simulink model "saved3"  (R2018b)
settings: Solver=VariableStepAuto  StartTime=0.0  StopTime=10.0  RelTol=1e-3
libraries: simulink x95, powerlib x8, powerlib_meascontrol x2
(part 5 of 6)

== system saved3/离散化半成品/PSMS2/PMSM dq ==
  u1 : Inport
  u2 : Inport  Port=2
  torE : Inport  Port=3
  Gain : Gain  Gain=1/2
  Gain1 : Gain  Gain=1/2
  Integrator{,1..3} (4 alike) : Integrator
  MATLAB Function : MATLAB Function  TreatAsAtomicUnit=on
  MATLAB Function1 : MATLAB Function  TreatAsAtomicUnit=on
  Sum : Sum  Inputs=|++
  角度增速测试 : simulink/Sources/Ramp  slope=0  start=0  InitialOutput=0
  i1 : Outport
  i2 : Outport  Port=2
  w : Outport  Port=3
  the : Outport  Port=4
  wires:
  MATLAB Function1/1(dw) -> Integrator2/1
  u1/1 -> Gain/1
  MATLAB Function/2(di2) -> Integrator1/1
  MATLAB Function/1(di1) -> Integrator/1
  Integrator/1 -> i1/1, MATLAB Function1/1(i1), MATLAB Function/3(i1)
  Integrator1/1 -> MATLAB Function/4(i2), MATLAB Function1/2(i2), i2/1
  torE/1 -> MATLAB Function1/4(torE)
  Gain/1 -> MATLAB Function/1(u1)
  u2/1 -> Gain1/1
  Gain1/1 -> MATLAB Function/2(u2)
  Integrator3/1 -> the/1
  Integrator2/1 -> Sum/1, MATLAB Function1/3(w), MATLAB Function/5(w), w/1
  Sum/1 -> Integrator3/1
  角度增速测试/1 -> Sum/2

== system saved3/离散化半成品/PSMS3/PMSM dq ==
  u1 : Inport
  u2 : Inport  Port=2
  torE : Inport  Port=3
  Gain : Gain  Gain=1/2
  Gain1 : Gain  Gain=1/2
  Integrator{,1..3} (4 alike) : Integrator
  MATLAB Function : MATLAB Function  TreatAsAtomicUnit=on
  MATLAB Function1 : MATLAB Function  TreatAsAtomicUnit=on
  Sum : Sum  Inputs=|++
  角度增速测试 : simulink/Sources/Ramp  slope=0  start=0  InitialOutput=0
  i1 : Outport
  i2 : Outport  Port=2
  w : Outport  Port=3
  the : Outport  Port=4
  wires:
  MATLAB Function1/1(dw) -> Integrator2/1
  u1/1 -> Gain/1
  MATLAB Function/2(di2) -> Integrator1/1
  MATLAB Function/1(di1) -> Integrator/1
  Integrator/1 -> i1/1, MATLAB Function1/1(i1), MATLAB Function/3(i1)
  Integrator1/1 -> MATLAB Function/4(i2), MATLAB Function1/2(i2), i2/1
  torE/1 -> MATLAB Function1/4(torE)
  Gain/1 -> MATLAB Function/1(u1)
  u2/1 -> Gain1/1
  Gain1/1 -> MATLAB Function/2(u2)
  Integrator3/1 -> the/1
  Integrator2/1 -> Sum/1, MATLAB Function1/3(w), MATLAB Function/5(w), w/1
  Sum/1 -> Integrator3/1
  角度增速测试/1 -> Sum/2

== system saved3/离散化半成品/Subsystem/电流采样 ==
  <Stator current is_a (A)> : Inport
  <Stator current is_b (A)> : Inport  Port=2
  <Stator current is_c (A)> : Inport  Port=3
  A/D转换 10KHz2 : MATLAB Function  TreatAsAtomicUnit=on  SystemSampleTime=1e-4
  A/D转换 10KHz3 : MATLAB Function  TreatAsAtomicUnit=on  SystemSampleTime=1e-4
  A/D转换 10KHz4 : MATLAB Function  TreatAsAtomicUnit=on  SystemSampleTime=1e-4
  Scope : Scope  NumInputPorts=3
  Sum1 : Sum  Inputs=|++
  Sum2 : Sum  Inputs=|++
  Sum3 : Sum  Inputs=|+-
  一阶滤波器40kHz1 : MATLAB Function  Commented=on  TreatAsAtomicUnit=on  SystemSampleTime=2.5e-5
  一阶滤波器40kHz2 : MATLAB Function  Commented=on  TreatAsAtomicUnit=on  SystemSampleTime=2.5e-5
  一阶滤波器40kHz3 : MATLAB Function  Commented=on  TreatAsAtomicUnit=on  SystemSampleTime=2.5e-5
  噪声 ia : simulink/Sources/Band-Limited White Noise  Cov=1e-7  Ts=1e-4  seed=[1]
  噪声 ib : simulink/Sources/Band-Limited White Noise  Cov=1e-7  Ts=1e-4  seed=[2]
  噪声 ic : simulink/Sources/Band-Limited White Noise  Cov=1e-7  Ts=1e-4  seed=[3]
  ia : Outport
  ib : Outport  Port=2
  ic : Outport  Port=3
  wires:
  Sum1/1 -> A/D转换 10KHz2/1(u)
  Sum2/1 -> A/D转换 10KHz3/1(u)
  Sum3/1 -> A/D转换 10KHz4/1(u)
  <Stator current is_b (A)>/1 -> Sum2/1
  <Stator current is_c (A)>/1 -> Sum3/1
  <Stator current is_a (A)>/1 -> Sum1/1
  A/D转换 10KHz2/1(y) -> Scope/1, ia/1
  A/D转换 10KHz3/1(y) -> Scope/2, ib/1
  A/D转换 10KHz4/1(y) -> Scope/3, ic/1
  噪声 ia/1 -> Sum1/2
  噪声 ic/1 -> Sum3/2
  噪声 ib/1 -> Sum2/2

== system saved3/离散化半成品/controller/方波注入 ==
  Constant2 : Constant  Value=0.5
  Gain11 : Gain  Gain=8
  Pulse Generator2 : DiscretePulseGenerator  PulseType=Time based  Period=1e-3  PulseWidth=50
  Sum4 : Sum  Inputs=|+-
  Out1 : Outport
  wires:
  Pulse Generator2/1 -> Sum4/1
  Sum4/1 -> Gain11/1
  Constant2/1 -> Sum4/2
  Gain11/1 -> Out1/1

== system saved3/离散化半成品/controller1/方波注入 ==
  Constant2 : Constant  Value=0.5
  Gain11 : Gain  Gain=8
  Pulse Generator2 : DiscretePulseGenerator  PulseType=Time based  Period=1e-3  PulseWidth=50
  Sum4 : Sum  Inputs=|+-
  Out1 : Outport
  wires:
  Pulse Generator2/1 -> Sum4/1
  Sum4/1 -> Gain11/1
  Constant2/1 -> Sum4/2
  Gain11/1 -> Out1/1

== system saved3/离散化半成品/controller2/方波注入 ==
  Constant2 : Constant  Value=0.5
  Gain11 : Gain  Gain=8
  Pulse Generator2 : DiscretePulseGenerator  PulseType=Time based  Period=1e-3  PulseWidth=50
  Sum4 : Sum  Inputs=|+-
  Out1 : Outport
  wires:
  Pulse Generator2/1 -> Sum4/1
  Sum4/1 -> Gain11/1
  Constant2/1 -> Sum4/2
  Gain11/1 -> Out1/1

== system saved3/离散化半成品/controller3/方波注入 ==
  Constant2 : Constant  Value=0.5
  Gain11 : Gain  Gain=8
  Pulse Generator2 : DiscretePulseGenerator  PulseType=Time based  Period=1e-3  PulseWidth=50
  Sum4 : Sum  Inputs=|+-
  Out1 : Outport
  wires:
  Pulse Generator2/1 -> Sum4/1
  Sum4/1 -> Gain11/1
  Constant2/1 -> Sum4/2
  Gain11/1 -> Out1/1

== system saved3/离散化半成品/current seperator/电流采样 ==
  <Stator current is_a (A)> : Inport
  <Stator current is_b (A)> : Inport  Port=2
  <Stator current is_c (A)> : Inport  Port=3
  A/D转换 10KHz2 : MATLAB Function  TreatAsAtomicUnit=on  SystemSampleTime=1e-4
  A/D转换 10KHz3 : MATLAB Function  TreatAsAtomicUnit=on  SystemSampleTime=1e-4
  A/D转换 10KHz4 : MATLAB Function  TreatAsAtomicUnit=on  SystemSampleTime=1e-4
  Scope : Scope  NumInputPorts=3
  Sum1 : Sum  Inputs=|++
  Sum2 : Sum  Inputs=|++
  Sum3 : Sum  Inputs=|+-
  噪声 ia : simulink/Sources/Band-Limited White Noise  Cov=1e-7  Ts=1e-4  seed=[1]
  噪声 ib : simulink/Sources/Band-Limited White Noise  Cov=1e-7  Ts=1e-4  seed=[2]
  噪声 ic : simulink/Sources/Band-Limited White Noise  Cov=1e-7  Ts=1e-4  seed=[3]
  ia : Outport
  ib : Outport  Port=2
  ic : Outport  Port=3
  wires:
  Sum1/1 -> A/D转换 10KHz2/1(u)
  Sum2/1 -> A/D转换 10KHz3/1(u)
  Sum3/1 -> A/D转换 10KHz4/1(u)
  <Stator current is_b (A)>/1 -> Sum2/1
  <Stator current is_c (A)>/1 -> Sum3/1
  <Stator current is_a (A)>/1 -> Sum1/1
  A/D转换 10KHz2/1(y) -> Scope/1, ia/1
  A/D转换 10KHz3/1(y) -> Scope/2, ib/1
  A/D转换 10KHz4/1(y) -> Scope/3, ic/1
  噪声 ia/1 -> Sum1/2
  噪声 ic/1 -> Sum3/2
  噪声 ib/1 -> Sum2/2

== system saved3/离散化半成品/current seperator/电流采样1 ==
  <Stator current is_a (A)> : Inport
  <Stator current is_b (A)> : Inport  Port=2
  <Stator current is_c (A)> : Inport  Port=3
  A/D转换 10KHz2 : MATLAB Function  TreatAsAtomicUnit=on  SystemSampleTime=1e-4
  A/D转换 10KHz3 : MATLAB Function  TreatAsAtomicUnit=on  SystemSampleTime=1e-4
  A/D转换 10KHz4 : MATLAB Function  TreatAsAtomicUnit=on  SystemSampleTime=1e-4
  Scope : Scope  NumInputPorts=3
  Sum1 : Sum  Inputs=|++
  Sum2 : Sum  Inputs=|++
  Sum3 : Sum  Inputs=|+-
  噪声 ia : simulink/Sources/Band-Limited White Noise  Cov=1e-7  Ts=1e-4  seed=[1]
  噪声 ib : simulink/Sources/Band-Limited White Noise  Cov=1e-7  Ts=1e-4  seed=[2]
  噪声 ic : simulink/Sources/Band-Limited White Noise  Cov=1e-7  Ts=1e-4  seed=[3]
  ia : Outport
  ib : Outport  Port=2
  ic : Outport  Port=3
  wires:
  Sum1/1 -> A/D转换 10KHz2/1(u)
  Sum2/1 -> A/D转换 10KHz3/1(u)
  Sum3/1 -> A/D转换 10KHz4/1(u)
  <Stator current is_b (A)>/1 -> Sum2/1
  <Stator current is_c (A)>/1 -> Sum3/1
  <Stator current is_a (A)>/1 -> Sum1/1
  A/D转换 10KHz2/1(y) -> Scope/1, ia/1
  A/D转换 10KHz3/1(y) -> Scope/2, ib/1
  A/D转换 10KHz4/1(y) -> Scope/3, ic/1
  噪声 ia/1 -> Sum1/2
  噪声 ic/1 -> Sum3/2
  噪声 ib/1 -> Sum2/2

== system saved3/离散化半成品/w estimater/Subsystem ==
  ua : Inport
  ub : Inport  Port=2
  ia : Inport  Port=3
  ib : Inport  Port=4
  1/Lm1 : Gain  Gain=1/1.2e-3
  1/Lm2 : Gain  Gain=1/1.2e-3
  Gain : Gain
  Gain1 : Gain
  Integrator : Integrator
  Integrator1 : Integrator
  PID Controller : simulink/Continuous/PID Controller  Controller=PID  Form=Parallel  TimeDomain=Continuous-time  SampleTime=-1  IntegratorMethod=Forward Euler  FilterMethod=Forward Euler  ControllerParametersSource=internal  P=10  I=10  D=1  UseFilter=on  N=100  TunerSelectOption=Transfer Function Based (PID Tuner App)  InitialConditionSource=internal  InitialConditionForIntegrator=0  InitialConditionForFilter=0  DifferentiatorICPrevScaledInput=0  ExternalReset=none  TrackingMode=off  Kt=1  LimitOutput=off  UpperSaturationLimit=inf  LowerSaturationLimit=-inf  LinearizeAsGain=on  AntiWindupMode=none  Kb=1  POutMin=[]  POutMax=[]  IOutMin=[]  IOutMax=[]  DOutMin=[]  DOutMax=[]  NOutMin=[]  NOutMax=[]  SumOutMin=[]  SumOutMax=[]  SaturationOutMin=[]  SaturationOutMax=[]  PParamMin=[]  PParamMax=[]  IParamMin=[]  IParamMax=[]  DParamMin=[]  DParamMax=[]  NParamMin=[]  NParamMax=[]  KbParamMin=[]  KbParamMax=[]  KtParamMin=[]  KtParamMax=[]  KbOutMin=[]  KbOutMax=[]  KtOutMin=[]  KtOutMax=[]  IntegratorOutMin=[]  IntegratorOutMax=[]  FilterOutMin=[]  FilterOutMax=[]  SumI1OutMin=[]  SumI1OutMax=[]  SumI2OutMin=[]  SumI2OutMax=[]  SumI3OutMin=[]  SumI3OutMax=[]  SumI4OutMin=[]  SumI4OutMax=[]  SumDOutMin=[]  SumDOutMax=[]  DifferentiatorOutMin=[]  DifferentiatorOutMax=[]  FilterDiffOutCoefMin=[]  FilterDiffOutCoefMax=[]  ReciprocalOutMin=[]  ReciprocalOutMax=[]  SumDenOutMin=[]  SumDenOutMax=[]  SumNumOutMin=[]  SumNumOutMax=[]  DivideOutMin=[]  DivideOutMax=[]  IntegratorContinuousStateAttributes=''  IntegratorStateMustResolveToSignalObject=off  IntegratorRTWStateStorageClass=Auto  FilterContinuousStateAttributes=''  FilterStateMustResolveToSignalObject=off  FilterRTWStateStorageClass=Auto  ParallelPVariant=InternalParameters  IdealPVariant=Disabled  IVariant=InternalParameters  DVariant=InternalParameters  IntegratorVariant=Continuous  SatVariant=Disabled  AWVariant=Passthrough  PCopyVariant=Disabled  TRVariant=Disabled  FdbkBlocksVariant=Forward  IdealPFdbkVariant=Disabled  SatFdbkVariant=Disabled  DerivativeFilterVariant=ContFilter  NVariant=InternalParameters  NCopyVariant=Disabled  FilterICVariant=InternalICsFilter  IntegratorICVariant=InternalICs  ExternalResetVariant=Disabled  TRSumVariant=Passthrough  SumFdbkVariant=Disabled  SumVariant=Sum_PID
  PID Controller1 : simulink/Continuous/PID Controller  Controller=PID  Form=Parallel  TimeDomain=Continuous-time  SampleTime=-1  IntegratorMethod=Forward Euler  FilterMethod=Forward Euler  ControllerParametersSource=internal  P=3  I=10  D=1  UseFilter=on  N=100  TunerSelectOption=Transfer Function Based (PID Tuner App)  InitialConditionSource=internal  InitialConditionForIntegrator=0  InitialConditionForFilter=0  DifferentiatorICPrevScaledInput=0  ExternalReset=none  TrackingMode=off  Kt=1  LimitOutput=off  UpperSaturationLimit=inf  LowerSaturationLimit=-inf  LinearizeAsGain=on  AntiWindupMode=none  Kb=1  POutMin=[]  POutMax=[]  IOutMin=[]  IOutMax=[]  DOutMin=[]  DOutMax=[]  NOutMin=[]  NOutMax=[]  SumOutMin=[]  SumOutMax=[]  SaturationOutMin=[]  SaturationOutMax=[]  PParamMin=[]  PParamMax=[]  IParamMin=[]  IParamMax=[]  DParamMin=[]  DParamMax=[]  NParamMin=[]  NParamMax=[]  KbParamMin=[]  KbParamMax=[]  KtParamMin=[]  KtParamMax=[]  KbOutMin=[]  KbOutMax=[]  KtOutMin=[]  KtOutMax=[]  IntegratorOutMin=[]  IntegratorOutMax=[]  FilterOutMin=[]  FilterOutMax=[]  SumI1OutMin=[]  SumI1OutMax=[]  SumI2OutMin=[]  SumI2OutMax=[]  SumI3OutMin=[]  SumI3OutMax=[]  SumI4OutMin=[]  SumI4OutMax=[]  SumDOutMin=[]  SumDOutMax=[]  DifferentiatorOutMin=[]  DifferentiatorOutMax=[]  FilterDiffOutCoefMin=[]  FilterDiffOutCoefMax=[]  ReciprocalOutMin=[]  ReciprocalOutMax=[]  SumDenOutMin=[]  SumDenOutMax=[]  SumNumOutMin=[]  SumNumOutMax=[]  DivideOutMin=[]  DivideOutMax=[]  IntegratorContinuousStateAttributes=''  IntegratorStateMustResolveToSignalObject=off  IntegratorRTWStateStorageClass=Auto  FilterContinuousStateAttributes=''  FilterStateMustResolveToSignalObject=off  FilterRTWStateStorageClass=Auto  ParallelPVariant=InternalParameters  IdealPVariant=Disabled  IVariant=InternalParameters  DVariant=InternalParameters  IntegratorVariant=Continuous  SatVariant=Disabled  AWVariant=Passthrough  PCopyVariant=Disabled  TRVariant=Disabled  FdbkBlocksVariant=Forward  IdealPFdbkVariant=Disabled  SatFdbkVariant=Disabled  DerivativeFilterVariant=ContFilter  NVariant=InternalParameters  NCopyVariant=Disabled  FilterICVariant=InternalICsFilter  IntegratorICVariant=InternalICs  ExternalResetVariant=Disabled  TRSumVariant=Passthrough  SumFdbkVariant=Disabled  SumVariant=Sum_PID
  R1 : Gain  Gain=0.1
  R2 : Gain  Gain=0.1
  Scope : Scope  NumInputPorts=2
  Scope1 : Scope  NumInputPorts=2
  Scope2 : Scope  NumInputPorts=2
  Sum : Sum  Inputs=|+-
  Sum1 : Sum  Inputs=++-
  Sum2 : Sum  Inputs=|+-
  Sum3 : Sum  Inputs=++-
  Ea : Outport
  Eb : Outport  Port=2
  wires:
  Sum/1 -> Gain1/1
  R1/1 -> Sum1/3
  Integrator/1 -> Scope2/2, Sum/2, R1/1
  Sum1/1 -> 1/Lm1/1
  1/Lm1/1 -> Integrator/1
  ua/1 -> Sum1/1
  ia/1 -> Scope2/1, Sum/1
  ib/1 -> Scope1/1, Sum2/1
  ub/1 -> Sum3/1
  Sum2/1 -> Gain/1
  1/Lm2/1 -> Integrator1/1
  R2/1 -> Sum3/3
  Sum3/1 -> 1/Lm2/1
  Integrator1/1 -> Sum2/2, Scope1/2, R2/1
  Gain/1 -> PID Controller1/1
  Gain1/1 -> PID Controller/1
  PID Controller1/1 -> Scope/2, Eb/1, Sum3/2
  PID Controller/1 -> Ea/1, Scope/1, Sum1/2

== system saved3/离散化半成品/w estimater/锁相环 ==
  cos : Inport
  sin : Inport  Port=2
  Constant : Constant  Value=0
  Cos : Trigonometry  Operator=cos
  Gain : Gain  Gain=-1
  Integrator2 : Integrator
  PID Controller : simulink/Continuous/PID Controller  Controller=PID  Form=Parallel  TimeDomain=Continuous-time  SampleTime=-1  IntegratorMethod=Forward Euler  FilterMethod=Forward Euler  ControllerParametersSource=internal  P=40  I=5000  D=0  UseFilter=on  N=100  TunerSelectOption=Transfer Function Based (PID Tuner App)  InitialConditionSource=internal  InitialConditionForIntegrator=0  InitialConditionForFilter=0  DifferentiatorICPrevScaledInput=0  ExternalReset=none  TrackingMode=off  Kt=1  LimitOutput=off  UpperSaturationLimit=inf  LowerSaturationLimit=-inf  LinearizeAsGain=on  AntiWindupMode=none  Kb=1  POutMin=[]  POutMax=[]  IOutMin=[]  IOutMax=[]  DOutMin=[]  DOutMax=[]  NOutMin=[]  NOutMax=[]  SumOutMin=[]  SumOutMax=[]  SaturationOutMin=[]  SaturationOutMax=[]  PParamMin=[]  PParamMax=[]  IParamMin=[]  IParamMax=[]  DParamMin=[]  DParamMax=[]  NParamMin=[]  NParamMax=[]  KbParamMin=[]  KbParamMax=[]  KtParamMin=[]  KtParamMax=[]  KbOutMin=[]  KbOutMax=[]  KtOutMin=[]  KtOutMax=[]  IntegratorOutMin=[]  IntegratorOutMax=[]  FilterOutMin=[]  FilterOutMax=[]  SumI1OutMin=[]  SumI1OutMax=[]  SumI2OutMin=[]  SumI2OutMax=[]  SumI3OutMin=[]  SumI3OutMax=[]  SumI4OutMin=[]  SumI4OutMax=[]  SumDOutMin=[]  SumDOutMax=[]  DifferentiatorOutMin=[]  DifferentiatorOutMax=[]  FilterDiffOutCoefMin=[]  FilterDiffOutCoefMax=[]  ReciprocalOutMin=[]  ReciprocalOutMax=[]  SumDenOutMin=[]  SumDenOutMax=[]  SumNumOutMin=[]  SumNumOutMax=[]  DivideOutMin=[]  DivideOutMax=[]  IntegratorContinuousStateAttributes=''  IntegratorStateMustResolveToSignalObject=off  IntegratorRTWStateStorageClass=Auto  FilterContinuousStateAttributes=''  FilterStateMustResolveToSignalObject=off  FilterRTWStateStorageClass=Auto  ParallelPVariant=InternalParameters  IdealPVariant=Disabled  IVariant=InternalParameters  DVariant=InternalParameters  IntegratorVariant=Continuous  SatVariant=Disabled  AWVariant=Passthrough  PCopyVariant=Disabled  TRVariant=Disabled  FdbkBlocksVariant=Forward  IdealPFdbkVariant=Disabled  SatFdbkVariant=Disabled  DerivativeFilterVariant=ContFilter  NVariant=InternalParameters  NCopyVariant=Disabled  FilterICVariant=InternalICsFilter  IntegratorICVariant=InternalICs  ExternalResetVariant=Disabled  TRSumVariant=Passthrough  SumFdbkVariant=Disabled  SumVariant=Sum_PID
  Product : Product
  Product1 : Product
  Saturation : Saturate  UpperLimit=500  LowerLimit=-500
  Scope : Scope
  Sin : Trigonometry
  Sum : Sum  Inputs=+-
  Sum1 : Sum  Inputs=|+-
  Transfer Fcn : TransferFcn  Numerator=[100]  Denominator=[1 100]
  Transfer Fcn1 : TransferFcn  Numerator=[100]  Denominator=[1 100]
  Transfer Fcn2 : TransferFcn  Numerator=[100]  Denominator=[1 100]
  we : Outport
  the : Outport  Port=2
  wires:
  cos/1 -> Transfer Fcn1/1
  Cos/1 -> Product1/2
  Product1/1 -> Sum/1
  Product/1 -> Sum/2
  Sin/1 -> Product/2
  Sum/1 -> PID Controller/1, Scope/1
  Integrator2/1 -> Sin/1, Cos/1, Sum1/1
  PID Controller/1 -> Saturation/1, Integrator2/1
  Transfer Fcn/1 -> we/1
  Sum1/1 -> the/1
  Constant/1 -> Sum1/2
  sin/1 -> Transfer Fcn2/1
  Gain/1 -> Product/1
  Saturation/1 -> Transfer Fcn/1
  Transfer Fcn1/1 -> Product1/1
  Transfer Fcn2/1 -> Gain/1

== system saved3/离散化半成品/w estimater1/Subsystem1 ==
  ua : Inport
  ub : Inport  Port=2
  ia : Inport  Port=3
  ib : Inport  Port=4
  1/Lm1 : Gain  Gain=1/1.2e-3
  1/Lm2 : Gain  Gain=1/1.2e-3
  Gain : Gain
  Gain1 : Gain
  Integrator : Integrator
  Integrator1 : Integrator
  PID Controller : simulink/Continuous/PID Controller  Controller=PID  Form=Parallel  TimeDomain=Continuous-time  SampleTime=-1  IntegratorMethod=Forward Euler  FilterMethod=Forward Euler  ControllerParametersSource=internal  P=10  I=10  D=1  UseFilter=on  N=100  TunerSelectOption=Transfer Function Based (PID Tuner App)  InitialConditionSource=internal  InitialConditionForIntegrator=0  InitialConditionForFilter=0  DifferentiatorICPrevScaledInput=0  ExternalReset=none  TrackingMode=off  Kt=1  LimitOutput=off  UpperSaturationLimit=inf  LowerSaturationLimit=-inf  LinearizeAsGain=on  AntiWindupMode=none  Kb=1  POutMin=[]  POutMax=[]  IOutMin=[]  IOutMax=[]  DOutMin=[]  DOutMax=[]  NOutMin=[]  NOutMax=[]  SumOutMin=[]  SumOutMax=[]  SaturationOutMin=[]  SaturationOutMax=[]  PParamMin=[]  PParamMax=[]  IParamMin=[]  IParamMax=[]  DParamMin=[]  DParamMax=[]  NParamMin=[]  NParamMax=[]  KbParamMin=[]  KbParamMax=[]  KtParamMin=[]  KtParamMax=[]  KbOutMin=[]  KbOutMax=[]  KtOutMin=[]  KtOutMax=[]  IntegratorOutMin=[]  IntegratorOutMax=[]  FilterOutMin=[]  FilterOutMax=[]  SumI1OutMin=[]  SumI1OutMax=[]  SumI2OutMin=[]  SumI2OutMax=[]  SumI3OutMin=[]  SumI3OutMax=[]  SumI4OutMin=[]  SumI4OutMax=[]  SumDOutMin=[]  SumDOutMax=[]  DifferentiatorOutMin=[]  DifferentiatorOutMax=[]  FilterDiffOutCoefMin=[]  FilterDiffOutCoefMax=[]  ReciprocalOutMin=[]  ReciprocalOutMax=[]  SumDenOutMin=[]  SumDenOutMax=[]  SumNumOutMin=[]  SumNumOutMax=[]  DivideOutMin=[]  DivideOutMax=[]  IntegratorContinuousStateAttributes=''  IntegratorStateMustResolveToSignalObject=off  IntegratorRTWStateStorageClass=Auto  FilterContinuousStateAttributes=''  FilterStateMustResolveToSignalObject=off  FilterRTWStateStorageClass=Auto  ParallelPVariant=InternalParameters  IdealPVariant=Disabled  IVariant=InternalParameters  DVariant=InternalParameters  IntegratorVariant=Continuous  SatVariant=Disabled  AWVariant=Passthrough  PCopyVariant=Disabled  TRVariant=Disabled  FdbkBlocksVariant=Forward  IdealPFdbkVariant=Disabled  SatFdbkVariant=Disabled  DerivativeFilterVariant=ContFilter  NVariant=InternalParameters  NCopyVariant=Disabled  FilterICVariant=InternalICsFilter  IntegratorICVariant=InternalICs  ExternalResetVariant=Disabled  TRSumVariant=Passthrough  SumFdbkVariant=Disabled  SumVariant=Sum_PID
  PID Controller1 : simulink/Continuous/PID Controller  Controller=PID  Form=Parallel  TimeDomain=Continuous-time  SampleTime=-1  IntegratorMethod=Forward Euler  FilterMethod=Forward Euler  ControllerParametersSource=internal  P=3  I=10  D=1  UseFilter=on  N=100  TunerSelectOption=Transfer Function Based (PID Tuner App)  InitialConditionSource=internal  InitialConditionForIntegrator=0  InitialConditionForFilter=0  DifferentiatorICPrevScaledInput=0  ExternalReset=none  TrackingMode=off  Kt=1  LimitOutput=off  UpperSaturationLimit=inf  LowerSaturationLimit=-inf  LinearizeAsGain=on  AntiWindupMode=none  Kb=1  POutMin=[]  POutMax=[]  IOutMin=[]  IOutMax=[]  DOutMin=[]  DOutMax=[]  NOutMin=[]  NOutMax=[]  SumOutMin=[]  SumOutMax=[]  SaturationOutMin=[]  SaturationOutMax=[]  PParamMin=[]  PParamMax=[]  IParamMin=[]  IParamMax=[]  DParamMin=[]  DParamMax=[]  NParamMin=[]  NParamMax=[]  KbParamMin=[]  KbParamMax=[]  KtParamMin=[]  KtParamMax=[]  KbOutMin=[]  KbOutMax=[]  KtOutMin=[]  KtOutMax=[]  IntegratorOutMin=[]  IntegratorOutMax=[]  FilterOutMin=[]  FilterOutMax=[]  SumI1OutMin=[]  SumI1OutMax=[]  SumI2OutMin=[]  SumI2OutMax=[]  SumI3OutMin=[]  SumI3OutMax=[]  SumI4OutMin=[]  SumI4OutMax=[]  SumDOutMin=[]  SumDOutMax=[]  DifferentiatorOutMin=[]  DifferentiatorOutMax=[]  FilterDiffOutCoefMin=[]  FilterDiffOutCoefMax=[]  ReciprocalOutMin=[]  ReciprocalOutMax=[]  SumDenOutMin=[]  SumDenOutMax=[]  SumNumOutMin=[]  SumNumOutMax=[]  DivideOutMin=[]  DivideOutMax=[]  IntegratorContinuousStateAttributes=''  IntegratorStateMustResolveToSignalObject=off  IntegratorRTWStateStorageClass=Auto  FilterContinuousStateAttributes=''  FilterStateMustResolveToSignalObject=off  FilterRTWStateStorageClass=Auto  ParallelPVariant=InternalParameters  IdealPVariant=Disabled  IVariant=InternalParameters  DVariant=InternalParameters  IntegratorVariant=Continuous  SatVariant=Disabled  AWVariant=Passthrough  PCopyVariant=Disabled  TRVariant=Disabled  FdbkBlocksVariant=Forward  IdealPFdbkVariant=Disabled  SatFdbkVariant=Disabled  DerivativeFilterVariant=ContFilter  NVariant=InternalParameters  NCopyVariant=Disabled  FilterICVariant=InternalICsFilter  IntegratorICVariant=InternalICs  ExternalResetVariant=Disabled  TRSumVariant=Passthrough  SumFdbkVariant=Disabled  SumVariant=Sum_PID
  R1 : Gain  Gain=0.1
  R2 : Gain  Gain=0.1
  Scope : Scope  NumInputPorts=2
  Scope1 : Scope  NumInputPorts=2
  Scope2 : Scope  NumInputPorts=2
  Sum : Sum  Inputs=|+-
  Sum1 : Sum  Inputs=++-
  Sum2 : Sum  Inputs=|+-
  Sum3 : Sum  Inputs=++-
  Ea : Outport
  Eb : Outport  Port=2
  wires:
  Sum/1 -> Gain1/1
  R1/1 -> Sum1/3
  Integrator/1 -> Scope2/2, Sum/2, R1/1
  Sum1/1 -> 1/Lm1/1
  1/Lm1/1 -> Integrator/1
  ua/1 -> Sum1/1
  ia/1 -> Scope2/1, Sum/1
  ib/1 -> Scope1/1, Sum2/1
  ub/1 -> Sum3/1
  Sum2/1 -> Gain/1
  1/Lm2/1 -> Integrator1/1
  R2/1 -> Sum3/3
  Sum3/1 -> 1/Lm2/1
  Integrator1/1 -> Sum2/2, Scope1/2, R2/1
  Gain/1 -> PID Controller1/1
  Gain1/1 -> PID Controller/1
  PID Controller1/1 -> Scope/2, Eb/1, Sum3/2
  PID Controller/1 -> Ea/1, Scope/1, Sum1/2

== system saved3/离散化半成品/w estimater1/锁相环1 ==
  cos : Inport
  sin : Inport  Port=2
  Constant : Constant  Value=0
  Cos : Trigonometry  Operator=cos
  Gain : Gain  Gain=-1
  Integrator2 : Integrator
  PID Controller : simulink/Continuous/PID Controller  Controller=PID  Form=Parallel  TimeDomain=Continuous-time  SampleTime=-1  IntegratorMethod=Forward Euler  FilterMethod=Forward Euler  ControllerParametersSource=internal  P=40  I=5000  D=0  UseFilter=on  N=100  TunerSelectOption=Transfer Function Based (PID Tuner App)  InitialConditionSource=internal  InitialConditionForIntegrator=0  InitialConditionForFilter=0  DifferentiatorICPrevScaledInput=0  ExternalReset=none  TrackingMode=off  Kt=1  LimitOutput=off  UpperSaturationLimit=inf  LowerSaturationLimit=-inf  LinearizeAsGain=on  AntiWindupMode=none  Kb=1  POutMin=[]  POutMax=[]  IOutMin=[]  IOutMax=[]  DOutMin=[]  DOutMax=[]  NOutMin=[]  NOutMax=[]  SumOutMin=[]  SumOutMax=[]  SaturationOutMin=[]  SaturationOutMax=[]  PParamMin=[]  PParamMax=[]  IParamMin=[]  IParamMax=[]  DParamMin=[]  DParamMax=[]  NParamMin=[]  NParamMax=[]  KbParamMin=[]  KbParamMax=[]  KtParamMin=[]  KtParamMax=[]  KbOutMin=[]  KbOutMax=[]  KtOutMin=[]  KtOutMax=[]  IntegratorOutMin=[]  IntegratorOutMax=[]  FilterOutMin=[]  FilterOutMax=[]  SumI1OutMin=[]  SumI1OutMax=[]  SumI2OutMin=[]  SumI2OutMax=[]  SumI3OutMin=[]  SumI3OutMax=[]  SumI4OutMin=[]  SumI4OutMax=[]  SumDOutMin=[]  SumDOutMax=[]  DifferentiatorOutMin=[]  DifferentiatorOutMax=[]  FilterDiffOutCoefMin=[]  FilterDiffOutCoefMax=[]  ReciprocalOutMin=[]  ReciprocalOutMax=[]  SumDenOutMin=[]  SumDenOutMax=[]  SumNumOutMin=[]  SumNumOutMax=[]  DivideOutMin=[]  DivideOutMax=[]  IntegratorContinuousStateAttributes=''  IntegratorStateMustResolveToSignalObject=off  IntegratorRTWStateStorageClass=Auto  FilterContinuousStateAttributes=''  FilterStateMustResolveToSignalObject=off  FilterRTWStateStorageClass=Auto  ParallelPVariant=InternalParameters  IdealPVariant=Disabled  IVariant=InternalParameters  DVariant=InternalParameters  IntegratorVariant=Continuous  SatVariant=Disabled  AWVariant=Passthrough  PCopyVariant=Disabled  TRVariant=Disabled  FdbkBlocksVariant=Forward  IdealPFdbkVariant=Disabled  SatFdbkVariant=Disabled  DerivativeFilterVariant=ContFilter  NVariant=InternalParameters  NCopyVariant=Disabled  FilterICVariant=InternalICsFilter  IntegratorICVariant=InternalICs  ExternalResetVariant=Disabled  TRSumVariant=Passthrough  SumFdbkVariant=Disabled  SumVariant=Sum_PID
  Product : Product
  Product1 : Product
  Saturation : Saturate  UpperLimit=500  LowerLimit=-500
  Scope : Scope
  Sin : Trigonometry
  Sum : Sum  Inputs=+-
  Sum1 : Sum  Inputs=|+-
  Transfer Fcn : TransferFcn  Numerator=[100]  Denominator=[1 100]
  Transfer Fcn1 : TransferFcn  Numerator=[100]  Denominator=[1 100]
  Transfer Fcn2 : TransferFcn  Numerator=[100]  Denominator=[1 100]
  we : Outport
  the : Outport  Port=2
  wires:
  cos/1 -> Transfer Fcn1/1
  Cos/1 -> Product1/2
  Product1/1 -> Sum/1
  Product/1 -> Sum/2
  Sin/1 -> Product/2
  Sum/1 -> PID Controller/1, Scope/1
  Integrator2/1 -> Sin/1, Cos/1, Sum1/1
  PID Controller/1 -> Saturation/1, Integrator2/1
  Transfer Fcn/1 -> we/1
  Sum1/1 -> the/1
  Constant/1 -> Sum1/2
  sin/1 -> Transfer Fcn2/1
  Gain/1 -> Product/1
  Saturation/1 -> Transfer Fcn/1
  Transfer Fcn1/1 -> Product1/1
  Transfer Fcn2/1 -> Gain/1

== system saved3/离散化半成品/w estimater2/Subsystem ==
  ua : Inport
  ub : Inport  Port=2
  ia : Inport  Port=3
  ib : Inport  Port=4
  1/Lm1 : Gain  Gain=1/1.2e-3
  1/Lm2 : Gain  Gain=1/1.2e-3
  Gain : Gain
  Gain1 : Gain
  Integrator : Integrator
  Integrator1 : Integrator
  PID Controller : simulink/Continuous/PID Controller  Controller=PID  Form=Parallel  TimeDomain=Continuous-time  SampleTime=-1  IntegratorMethod=Forward Euler  FilterMethod=Forward Euler  ControllerParametersSource=internal  P=10  I=10  D=1  UseFilter=on  N=100  TunerSelectOption=Transfer Function Based (PID Tuner App)  InitialConditionSource=internal  InitialConditionForIntegrator=0  InitialConditionForFilter=0  DifferentiatorICPrevScaledInput=0  ExternalReset=none  TrackingMode=off  Kt=1  LimitOutput=off  UpperSaturationLimit=inf  LowerSaturationLimit=-inf  LinearizeAsGain=on  AntiWindupMode=none  Kb=1  POutMin=[]  POutMax=[]  IOutMin=[]  IOutMax=[]  DOutMin=[]  DOutMax=[]  NOutMin=[]  NOutMax=[]  SumOutMin=[]  SumOutMax=[]  SaturationOutMin=[]  SaturationOutMax=[]  PParamMin=[]  PParamMax=[]  IParamMin=[]  IParamMax=[]  DParamMin=[]  DParamMax=[]  NParamMin=[]  NParamMax=[]  KbParamMin=[]  KbParamMax=[]  KtParamMin=[]  KtParamMax=[]  KbOutMin=[]  KbOutMax=[]  KtOutMin=[]  KtOutMax=[]  IntegratorOutMin=[]  IntegratorOutMax=[]  FilterOutMin=[]  FilterOutMax=[]  SumI1OutMin=[]  SumI1OutMax=[]  SumI2OutMin=[]  SumI2OutMax=[]  SumI3OutMin=[]  SumI3OutMax=[]  SumI4OutMin=[]  SumI4OutMax=[]  SumDOutMin=[]  SumDOutMax=[]  DifferentiatorOutMin=[]  DifferentiatorOutMax=[]  FilterDiffOutCoefMin=[]  FilterDiffOutCoefMax=[]  ReciprocalOutMin=[]  ReciprocalOutMax=[]  SumDenOutMin=[]  SumDenOutMax=[]  SumNumOutMin=[]  SumNumOutMax=[]  DivideOutMin=[]  DivideOutMax=[]  IntegratorContinuousStateAttributes=''  IntegratorStateMustResolveToSignalObject=off  IntegratorRTWStateStorageClass=Auto  FilterContinuousStateAttributes=''  FilterStateMustResolveToSignalObject=off  FilterRTWStateStorageClass=Auto  ParallelPVariant=InternalParameters  IdealPVariant=Disabled  IVariant=InternalParameters  DVariant=InternalParameters  IntegratorVariant=Continuous  SatVariant=Disabled  AWVariant=Passthrough  PCopyVariant=Disabled  TRVariant=Disabled  FdbkBlocksVariant=Forward  IdealPFdbkVariant=Disabled  SatFdbkVariant=Disabled  DerivativeFilterVariant=ContFilter  NVariant=InternalParameters  NCopyVariant=Disabled  FilterICVariant=InternalICsFilter  IntegratorICVariant=InternalICs  ExternalResetVariant=Disabled  TRSumVariant=Passthrough  SumFdbkVariant=Disabled  SumVariant=Sum_PID
  PID Controller1 : simulink/Continuous/PID Controller  Controller=PID  Form=Parallel  TimeDomain=Continuous-time  SampleTime=-1  IntegratorMethod=Forward Euler  FilterMethod=Forward Euler  ControllerParametersSource=internal  P=3  I=10  D=1  UseFilter=on  N=100  TunerSelectOption=Transfer Function Based (PID Tuner App)  InitialConditionSource=internal  InitialConditionForIntegrator=0  InitialConditionForFilter=0  DifferentiatorICPrevScaledInput=0  ExternalReset=none  TrackingMode=off  Kt=1  LimitOutput=off  UpperSaturationLimit=inf  LowerSaturationLimit=-inf  LinearizeAsGain=on  AntiWindupMode=none  Kb=1  POutMin=[]  POutMax=[]  IOutMin=[]  IOutMax=[]  DOutMin=[]  DOutMax=[]  NOutMin=[]  NOutMax=[]  SumOutMin=[]  SumOutMax=[]  SaturationOutMin=[]  SaturationOutMax=[]  PParamMin=[]  PParamMax=[]  IParamMin=[]  IParamMax=[]  DParamMin=[]  DParamMax=[]  NParamMin=[]  NParamMax=[]  KbParamMin=[]  KbParamMax=[]  KtParamMin=[]  KtParamMax=[]  KbOutMin=[]  KbOutMax=[]  KtOutMin=[]  KtOutMax=[]  IntegratorOutMin=[]  IntegratorOutMax=[]  FilterOutMin=[]  FilterOutMax=[]  SumI1OutMin=[]  SumI1OutMax=[]  SumI2OutMin=[]  SumI2OutMax=[]  SumI3OutMin=[]  SumI3OutMax=[]  SumI4OutMin=[]  SumI4OutMax=[]  SumDOutMin=[]  SumDOutMax=[]  DifferentiatorOutMin=[]  DifferentiatorOutMax=[]  FilterDiffOutCoefMin=[]  FilterDiffOutCoefMax=[]  ReciprocalOutMin=[]  ReciprocalOutMax=[]  SumDenOutMin=[]  SumDenOutMax=[]  SumNumOutMin=[]  SumNumOutMax=[]  DivideOutMin=[]  DivideOutMax=[]  IntegratorContinuousStateAttributes=''  IntegratorStateMustResolveToSignalObject=off  IntegratorRTWStateStorageClass=Auto  FilterContinuousStateAttributes=''  FilterStateMustResolveToSignalObject=off  FilterRTWStateStorageClass=Auto  ParallelPVariant=InternalParameters  IdealPVariant=Disabled  IVariant=InternalParameters  DVariant=InternalParameters  IntegratorVariant=Continuous  SatVariant=Disabled  AWVariant=Passthrough  PCopyVariant=Disabled  TRVariant=Disabled  FdbkBlocksVariant=Forward  IdealPFdbkVariant=Disabled  SatFdbkVariant=Disabled  DerivativeFilterVariant=ContFilter  NVariant=InternalParameters  NCopyVariant=Disabled  FilterICVariant=InternalICsFilter  IntegratorICVariant=InternalICs  ExternalResetVariant=Disabled  TRSumVariant=Passthrough  SumFdbkVariant=Disabled  SumVariant=Sum_PID
  R1 : Gain  Gain=0.1
  R2 : Gain  Gain=0.1
  Scope : Scope  NumInputPorts=2
  Scope1 : Scope  NumInputPorts=2
  Scope2 : Scope  NumInputPorts=2
  Sum : Sum  Inputs=|+-
  Sum1 : Sum  Inputs=++-
  Sum2 : Sum  Inputs=|+-
  Sum3 : Sum  Inputs=++-
  Ea : Outport
  Eb : Outport  Port=2
  wires:
  Sum/1 -> Gain1/1
  R1/1 -> Sum1/3
  Integrator/1 -> Scope2/2, Sum/2, R1/1
  Sum1/1 -> 1/Lm1/1
  1/Lm1/1 -> Integrator/1
  ua/1 -> Sum1/1
  ia/1 -> Scope2/1, Sum/1
  ib/1 -> Scope1/1, Sum2/1
  ub/1 -> Sum3/1
  Sum2/1 -> Gain/1
  1/Lm2/1 -> Integrator1/1
  R2/1 -> Sum3/3
  Sum3/1 -> 1/Lm2/1
  Integrator1/1 -> Sum2/2, Scope1/2, R2/1
  Gain/1 -> PID Controller1/1
  Gain1/1 -> PID Controller/1
  PID Controller1/1 -> Scope/2, Eb/1, Sum3/2
  PID Controller/1 -> Ea/1, Scope/1, Sum1/2

== system saved3/离散化半成品/w estimater2/锁相环 ==
  cos : Inport
  sin : Inport  Port=2
  Constant : Constant  Value=0
  Cos : Trigonometry  Operator=cos
  Gain : Gain  Gain=-1
  Integrator2 : Integrator
  PID Controller : simulink/Continuous/PID Controller  Controller=PID  Form=Parallel  TimeDomain=Continuous-time  SampleTime=-1  IntegratorMethod=Forward Euler  FilterMethod=Forward Euler  ControllerParametersSource=internal  P=40  I=5000  D=0  UseFilter=on  N=100  TunerSelectOption=Transfer Function Based (PID Tuner App)  InitialConditionSource=internal  InitialConditionForIntegrator=0  InitialConditionForFilter=0  DifferentiatorICPrevScaledInput=0  ExternalReset=none  TrackingMode=off  Kt=1  LimitOutput=off  UpperSaturationLimit=inf  LowerSaturationLimit=-inf  LinearizeAsGain=on  AntiWindupMode=none  Kb=1  POutMin=[]  POutMax=[]  IOutMin=[]  IOutMax=[]  DOutMin=[]  DOutMax=[]  NOutMin=[]  NOutMax=[]  SumOutMin=[]  SumOutMax=[]  SaturationOutMin=[]  SaturationOutMax=[]  PParamMin=[]  PParamMax=[]  IParamMin=[]  IParamMax=[]  DParamMin=[]  DParamMax=[]  NParamMin=[]  NParamMax=[]  KbParamMin=[]  KbParamMax=[]  KtParamMin=[]  KtParamMax=[]  KbOutMin=[]  KbOutMax=[]  KtOutMin=[]  KtOutMax=[]  IntegratorOutMin=[]  IntegratorOutMax=[]  FilterOutMin=[]  FilterOutMax=[]  SumI1OutMin=[]  SumI1OutMax=[]  SumI2OutMin=[]  SumI2OutMax=[]  SumI3OutMin=[]  SumI3OutMax=[]  SumI4OutMin=[]  SumI4OutMax=[]  SumDOutMin=[]  SumDOutMax=[]  DifferentiatorOutMin=[]  DifferentiatorOutMax=[]  FilterDiffOutCoefMin=[]  FilterDiffOutCoefMax=[]  ReciprocalOutMin=[]  ReciprocalOutMax=[]  SumDenOutMin=[]  SumDenOutMax=[]  SumNumOutMin=[]  SumNumOutMax=[]  DivideOutMin=[]  DivideOutMax=[]  IntegratorContinuousStateAttributes=''  IntegratorStateMustResolveToSignalObject=off  IntegratorRTWStateStorageClass=Auto  FilterContinuousStateAttributes=''  FilterStateMustResolveToSignalObject=off  FilterRTWStateStorageClass=Auto  ParallelPVariant=InternalParameters  IdealPVariant=Disabled  IVariant=InternalParameters  DVariant=InternalParameters  IntegratorVariant=Continuous  SatVariant=Disabled  AWVariant=Passthrough  PCopyVariant=Disabled  TRVariant=Disabled  FdbkBlocksVariant=Forward  IdealPFdbkVariant=Disabled  SatFdbkVariant=Disabled  DerivativeFilterVariant=ContFilter  NVariant=InternalParameters  NCopyVariant=Disabled  FilterICVariant=InternalICsFilter  IntegratorICVariant=InternalICs  ExternalResetVariant=Disabled  TRSumVariant=Passthrough  SumFdbkVariant=Disabled  SumVariant=Sum_PID
  Product : Product
  Product1 : Product
  Saturation : Saturate  UpperLimit=500  LowerLimit=-500
  Scope : Scope
  Sin : Trigonometry
  Sum : Sum  Inputs=+-
  Sum1 : Sum  Inputs=|+-
  Transfer Fcn : TransferFcn  Numerator=[100]  Denominator=[1 100]
  Transfer Fcn1 : TransferFcn  Numerator=[100]  Denominator=[1 100]
  Transfer Fcn2 : TransferFcn  Numerator=[100]  Denominator=[1 100]
  we : Outport
  the : Outport  Port=2
  wires:
  cos/1 -> Transfer Fcn1/1
  Cos/1 -> Product1/2
  Product1/1 -> Sum/1
  Product/1 -> Sum/2
  Sin/1 -> Product/2
  Sum/1 -> PID Controller/1, Scope/1
  Integrator2/1 -> Sin/1, Cos/1, Sum1/1
  PID Controller/1 -> Saturation/1, Integrator2/1
  Transfer Fcn/1 -> we/1
  Sum1/1 -> the/1
  Constant/1 -> Sum1/2
  sin/1 -> Transfer Fcn2/1
  Gain/1 -> Product/1
  Saturation/1 -> Transfer Fcn/1
  Transfer Fcn1/1 -> Product1/1
  Transfer Fcn2/1 -> Gain/1

== system saved3/离散化半成品/w estimater3/Subsystem ==
  ua : Inport
  ub : Inport  Port=2
  ia : Inport  Port=3
  ib : Inport  Port=4
  1/Lm1 : Gain  Gain=1/1.2e-3
  1/Lm2 : Gain  Gain=1/1.2e-3
  Gain : Gain
  Gain1 : Gain
  Integrator : Integrator
  Integrator1 : Integrator
  PID Controller : simulink/Continuous/PID Controller  Controller=PID  Form=Parallel  TimeDomain=Continuous-time  SampleTime=-1  IntegratorMethod=Forward Euler  FilterMethod=Forward Euler  ControllerParametersSource=internal  P=10  I=10  D=1  UseFilter=on  N=100  TunerSelectOption=Transfer Function Based (PID Tuner App)  InitialConditionSource=internal  InitialConditionForIntegrator=0  InitialConditionForFilter=0  DifferentiatorICPrevScaledInput=0  ExternalReset=none  TrackingMode=off  Kt=1  LimitOutput=off  UpperSaturationLimit=inf  LowerSaturationLimit=-inf  LinearizeAsGain=on  AntiWindupMode=none  Kb=1  POutMin=[]  POutMax=[]  IOutMin=[]  IOutMax=[]  DOutMin=[]  DOutMax=[]  NOutMin=[]  NOutMax=[]  SumOutMin=[]  SumOutMax=[]  SaturationOutMin=[]  SaturationOutMax=[]  PParamMin=[]  PParamMax=[]  IParamMin=[]  IParamMax=[]  DParamMin=[]  DParamMax=[]  NParamMin=[]  NParamMax=[]  KbParamMin=[]  KbParamMax=[]  KtParamMin=[]  KtParamMax=[]  KbOutMin=[]  KbOutMax=[]  KtOutMin=[]  KtOutMax=[]  IntegratorOutMin=[]  IntegratorOutMax=[]  FilterOutMin=[]  FilterOutMax=[]  SumI1OutMin=[]  SumI1OutMax=[]  SumI2OutMin=[]  SumI2OutMax=[]  SumI3OutMin=[]  SumI3OutMax=[]  SumI4OutMin=[]  SumI4OutMax=[]  SumDOutMin=[]  SumDOutMax=[]  DifferentiatorOutMin=[]  DifferentiatorOutMax=[]  FilterDiffOutCoefMin=[]  FilterDiffOutCoefMax=[]  ReciprocalOutMin=[]  ReciprocalOutMax=[]  SumDenOutMin=[]  SumDenOutMax=[]  SumNumOutMin=[]  SumNumOutMax=[]  DivideOutMin=[]  DivideOutMax=[]  IntegratorContinuousStateAttributes=''  IntegratorStateMustResolveToSignalObject=off  IntegratorRTWStateStorageClass=Auto  FilterContinuousStateAttributes=''  FilterStateMustResolveToSignalObject=off  FilterRTWStateStorageClass=Auto  ParallelPVariant=InternalParameters  IdealPVariant=Disabled  IVariant=InternalParameters  DVariant=InternalParameters  IntegratorVariant=Continuous  SatVariant=Disabled  AWVariant=Passthrough  PCopyVariant=Disabled  TRVariant=Disabled  FdbkBlocksVariant=Forward  IdealPFdbkVariant=Disabled  SatFdbkVariant=Disabled  DerivativeFilterVariant=ContFilter  NVariant=InternalParameters  NCopyVariant=Disabled  FilterICVariant=InternalICsFilter  IntegratorICVariant=InternalICs  ExternalResetVariant=Disabled  TRSumVariant=Passthrough  SumFdbkVariant=Disabled  SumVariant=Sum_PID
  PID Controller1 : simulink/Continuous/PID Controller  Controller=PID  Form=Parallel  TimeDomain=Continuous-time  SampleTime=-1  IntegratorMethod=Forward Euler  FilterMethod=Forward Euler  ControllerParametersSource=internal  P=3  I=10  D=1  UseFilter=on  N=100  TunerSelectOption=Transfer Function Based (PID Tuner App)  InitialConditionSource=internal  InitialConditionForIntegrator=0  InitialConditionForFilter=0  DifferentiatorICPrevScaledInput=0  ExternalReset=none  TrackingMode=off  Kt=1  LimitOutput=off  UpperSaturationLimit=inf  LowerSaturationLimit=-inf  LinearizeAsGain=on  AntiWindupMode=none  Kb=1  POutMin=[]  POutMax=[]  IOutMin=[]  IOutMax=[]  DOutMin=[]  DOutMax=[]  NOutMin=[]  NOutMax=[]  SumOutMin=[]  SumOutMax=[]  SaturationOutMin=[]  SaturationOutMax=[]  PParamMin=[]  PParamMax=[]  IParamMin=[]  IParamMax=[]  DParamMin=[]  DParamMax=[]  NParamMin=[]  NParamMax=[]  KbParamMin=[]  KbParamMax=[]  KtParamMin=[]  KtParamMax=[]  KbOutMin=[]  KbOutMax=[]  KtOutMin=[]  KtOutMax=[]  IntegratorOutMin=[]  IntegratorOutMax=[]  FilterOutMin=[]  FilterOutMax=[]  SumI1OutMin=[]  SumI1OutMax=[]  SumI2OutMin=[]  SumI2OutMax=[]  SumI3OutMin=[]  SumI3OutMax=[]  SumI4OutMin=[]  SumI4OutMax=[]  SumDOutMin=[]  SumDOutMax=[]  DifferentiatorOutMin=[]  DifferentiatorOutMax=[]  FilterDiffOutCoefMin=[]  FilterDiffOutCoefMax=[]  ReciprocalOutMin=[]  ReciprocalOutMax=[]  SumDenOutMin=[]  SumDenOutMax=[]  SumNumOutMin=[]  SumNumOutMax=[]  DivideOutMin=[]  DivideOutMax=[]  IntegratorContinuousStateAttributes=''  IntegratorStateMustResolveToSignalObject=off  IntegratorRTWStateStorageClass=Auto  FilterContinuousStateAttributes=''  FilterStateMustResolveToSignalObject=off  FilterRTWStateStorageClass=Auto  ParallelPVariant=InternalParameters  IdealPVariant=Disabled  IVariant=InternalParameters  DVariant=InternalParameters  IntegratorVariant=Continuous  SatVariant=Disabled  AWVariant=Passthrough  PCopyVariant=Disabled  TRVariant=Disabled  FdbkBlocksVariant=Forward  IdealPFdbkVariant=Disabled  SatFdbkVariant=Disabled  DerivativeFilterVariant=ContFilter  NVariant=InternalParameters  NCopyVariant=Disabled  FilterICVariant=InternalICsFilter  IntegratorICVariant=InternalICs  ExternalResetVariant=Disabled  TRSumVariant=Passthrough  SumFdbkVariant=Disabled  SumVariant=Sum_PID
  R1 : Gain  Gain=0.1
  R2 : Gain  Gain=0.1
  Scope : Scope  NumInputPorts=2
  Scope1 : Scope  NumInputPorts=2
  Scope2 : Scope  NumInputPorts=2
  Sum : Sum  Inputs=|+-
  Sum1 : Sum  Inputs=++-
  Sum2 : Sum  Inputs=|+-
  Sum3 : Sum  Inputs=++-
  Ea : Outport
  Eb : Outport  Port=2
  wires:
  Sum/1 -> Gain1/1
  R1/1 -> Sum1/3
  Integrator/1 -> Scope2/2, Sum/2, R1/1
  Sum1/1 -> 1/Lm1/1
  1/Lm1/1 -> Integrator/1
  ua/1 -> Sum1/1
  ia/1 -> Scope2/1, Sum/1
  ib/1 -> Scope1/1, Sum2/1
  ub/1 -> Sum3/1
  Sum2/1 -> Gain/1
  1/Lm2/1 -> Integrator1/1
  R2/1 -> Sum3/3
  Sum3/1 -> 1/Lm2/1
  Integrator1/1 -> Sum2/2, Scope1/2, R2/1
  Gain/1 -> PID Controller1/1
  Gain1/1 -> PID Controller/1
  PID Controller1/1 -> Scope/2, Eb/1, Sum3/2
  PID Controller/1 -> Ea/1, Scope/1, Sum1/2

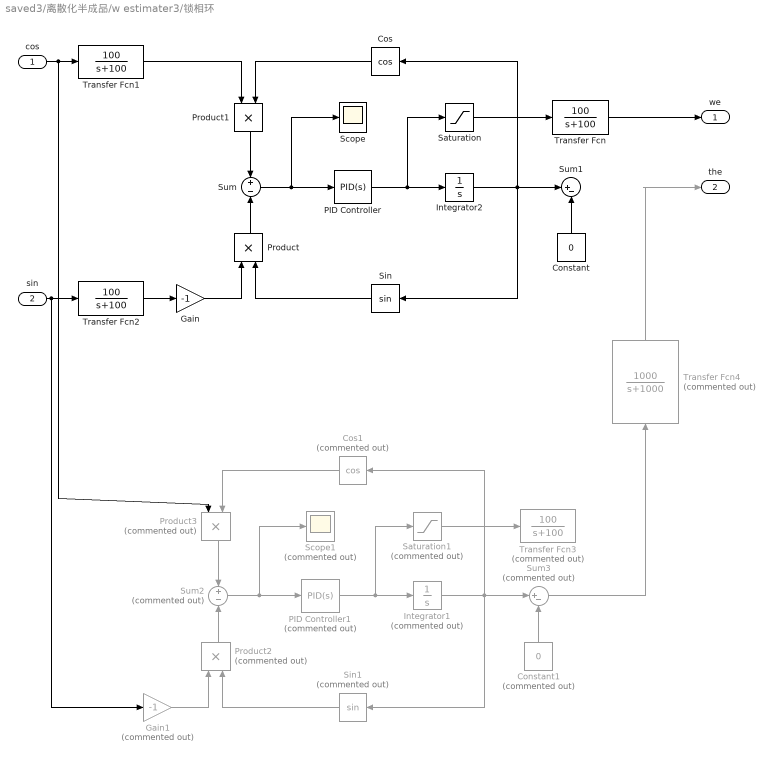
== system saved3/离散化半成品/w estimater3/锁相环 ==
  cos : Inport
  sin : Inport  Port=2
  Constant : Constant  Value=0
  Constant1 : Constant  Commented=on  Value=0
  Cos : Trigonometry  Operator=cos
  Cos1 : Trigonometry  Commented=on  Operator=cos
  Gain : Gain  Gain=-1
  Gain1 : Gain  Commented=on  Gain=-1
  Integrator1 : Integrator  Commented=on
  Integrator2 : Integrator
  PID Controller : simulink/Continuous/PID Controller  Controller=PID  Form=Parallel  TimeDomain=Continuous-time  SampleTime=-1  IntegratorMethod=Forward Euler  FilterMethod=Forward Euler  ControllerParametersSource=internal  P=40  I=5000  D=0  UseFilter=on  N=100  TunerSelectOption=Transfer Function Based (PID Tuner App)  InitialConditionSource=internal  InitialConditionForIntegrator=0  InitialConditionForFilter=0  DifferentiatorICPrevScaledInput=0  ExternalReset=none  TrackingMode=off  Kt=1  LimitOutput=off  UpperSaturationLimit=inf  LowerSaturationLimit=-inf  LinearizeAsGain=on  AntiWindupMode=none  Kb=1  POutMin=[]  POutMax=[]  IOutMin=[]  IOutMax=[]  DOutMin=[]  DOutMax=[]  NOutMin=[]  NOutMax=[]  SumOutMin=[]  SumOutMax=[]  SaturationOutMin=[]  SaturationOutMax=[]  PParamMin=[]  PParamMax=[]  IParamMin=[]  IParamMax=[]  DParamMin=[]  DParamMax=[]  NParamMin=[]  NParamMax=[]  KbParamMin=[]  KbParamMax=[]  KtParamMin=[]  KtParamMax=[]  KbOutMin=[]  KbOutMax=[]  KtOutMin=[]  KtOutMax=[]  IntegratorOutMin=[]  IntegratorOutMax=[]  FilterOutMin=[]  FilterOutMax=[]  SumI1OutMin=[]  SumI1OutMax=[]  SumI2OutMin=[]  SumI2OutMax=[]  SumI3OutMin=[]  SumI3OutMax=[]  SumI4OutMin=[]  SumI4OutMax=[]  SumDOutMin=[]  SumDOutMax=[]  DifferentiatorOutMin=[]  DifferentiatorOutMax=[]  FilterDiffOutCoefMin=[]  FilterDiffOutCoefMax=[]  ReciprocalOutMin=[]  ReciprocalOutMax=[]  SumDenOutMin=[]  SumDenOutMax=[]  SumNumOutMin=[]  SumNumOutMax=[]  DivideOutMin=[]  DivideOutMax=[]  IntegratorContinuousStateAttributes=''  IntegratorStateMustResolveToSignalObject=off  IntegratorRTWStateStorageClass=Auto  FilterContinuousStateAttributes=''  FilterStateMustResolveToSignalObject=off  FilterRTWStateStorageClass=Auto  ParallelPVariant=InternalParameters  IdealPVariant=Disabled  IVariant=InternalParameters  DVariant=InternalParameters  IntegratorVariant=Continuous  SatVariant=Disabled  AWVariant=Passthrough  PCopyVariant=Disabled  TRVariant=Disabled  FdbkBlocksVariant=Forward  IdealPFdbkVariant=Disabled  SatFdbkVariant=Disabled  DerivativeFilterVariant=ContFilter  NVariant=InternalParameters  NCopyVariant=Disabled  FilterICVariant=InternalICsFilter  IntegratorICVariant=InternalICs  ExternalResetVariant=Disabled  TRSumVariant=Passthrough  SumFdbkVariant=Disabled  SumVariant=Sum_PID
  PID Controller1 : simulink/Continuous/PID Controller  Commented=on  Controller=PID  Form=Parallel  TimeDomain=Continuous-time  SampleTime=-1  IntegratorMethod=Forward Euler  FilterMethod=Forward Euler  ControllerParametersSource=internal  P=400  I=50000  D=0  UseFilter=on  N=100  TunerSelectOption=Transfer Function Based (PID Tuner App)  InitialConditionSource=internal  InitialConditionForIntegrator=0  InitialConditionForFilter=0  DifferentiatorICPrevScaledInput=0  ExternalReset=none  TrackingMode=off  Kt=1  LimitOutput=off  UpperSaturationLimit=inf  LowerSaturationLimit=-inf  LinearizeAsGain=on  AntiWindupMode=none  Kb=1  POutMin=[]  POutMax=[]  IOutMin=[]  IOutMax=[]  DOutMin=[]  DOutMax=[]  NOutMin=[]  NOutMax=[]  SumOutMin=[]  SumOutMax=[]  SaturationOutMin=[]  SaturationOutMax=[]  PParamMin=[]  PParamMax=[]  IParamMin=[]  IParamMax=[]  DParamMin=[]  DParamMax=[]  NParamMin=[]  NParamMax=[]  KbParamMin=[]  KbParamMax=[]  KtParamMin=[]  KtParamMax=[]  KbOutMin=[]  KbOutMax=[]  KtOutMin=[]  KtOutMax=[]  IntegratorOutMin=[]  IntegratorOutMax=[]  FilterOutMin=[]  FilterOutMax=[]  SumI1OutMin=[]  SumI1OutMax=[]  SumI2OutMin=[]  SumI2OutMax=[]  SumI3OutMin=[]  SumI3OutMax=[]  SumI4OutMin=[]  SumI4OutMax=[]  SumDOutMin=[]  SumDOutMax=[]  DifferentiatorOutMin=[]  DifferentiatorOutMax=[]  FilterDiffOutCoefMin=[]  FilterDiffOutCoefMax=[]  ReciprocalOutMin=[]  ReciprocalOutMax=[]  SumDenOutMin=[]  SumDenOutMax=[]  SumNumOutMin=[]  SumNumOutMax=[]  DivideOutMin=[]  DivideOutMax=[]  IntegratorContinuousStateAttributes=''  IntegratorStateMustResolveToSignalObject=off  IntegratorRTWStateStorageClass=Auto  FilterContinuousStateAttributes=''  FilterStateMustResolveToSignalObject=off  FilterRTWStateStorageClass=Auto  ParallelPVariant=InternalParameters  IdealPVariant=Disabled  IVariant=InternalParameters  DVariant=InternalParameters  IntegratorVariant=Continuous  SatVariant=Disabled  AWVariant=Passthrough  PCopyVariant=Disabled  TRVariant=Disabled  FdbkBlocksVariant=Forward  IdealPFdbkVariant=Disabled  SatFdbkVariant=Disabled  DerivativeFilterVariant=ContFilter  NVariant=InternalParameters  NCopyVariant=Disabled  FilterICVariant=InternalICsFilter  IntegratorICVariant=InternalICs  ExternalResetVariant=Disabled  TRSumVariant=Passthrough  SumFdbkVariant=Disabled  SumVariant=Sum_PID
  Product : Product
  Product1 : Product
  Product2 : Product  Commented=on
  Product3 : Product  Commented=on
  Saturation : Saturate  UpperLimit=500  LowerLimit=-500
  Saturation1 : Saturate  Commented=on  UpperLimit=500  LowerLimit=-500
  Scope : Scope
  Scope1 : Scope  Commented=on
  Sin : Trigonometry
  Sin1 : Trigonometry  Commented=on
  Sum : Sum  Inputs=+-
  Sum1 : Sum  Inputs=|+-
  Sum2 : Sum  Commented=on  Inputs=+-
  Sum3 : Sum  Commented=on  Inputs=|+-
  Transfer Fcn : TransferFcn  Numerator=[100]  Denominator=[1 100]
  Transfer Fcn1 : TransferFcn  Numerator=[100]  Denominator=[1 100]
  Transfer Fcn2 : TransferFcn  Numerator=[100]  Denominator=[1 100]
  Transfer Fcn3 : TransferFcn  Commented=on  Numerator=[100]  Denominator=[1 100]
  Transfer Fcn4 : TransferFcn  Commented=on  Numerator=[1000]  Denominator=[1 1000]
  we : Outport
  the : Outport  Port=2
  wires:
  Cos/1 -> Product1/2
  Product1/1 -> Sum/1
  Product/1 -> Sum/2
  Sin/1 -> Product/2
  Sum/1 -> PID Controller/1, Scope/1
  Integrator2/1 -> Sin/1, Cos/1, Sum1/1
  PID Controller/1 -> Saturation/1, Integrator2/1
  Transfer Fcn/1 -> we/1
  Constant/1 -> Sum1/2
  Gain/1 -> Product/1
  Saturation/1 -> Transfer Fcn/1
  Transfer Fcn1/1 -> Product1/1
  Transfer Fcn2/1 -> Gain/1
  sin/1 -> Gain1/1, Transfer Fcn2/1
  Saturation1/1 -> Transfer Fcn3/1
  Gain1/1 -> Product2/1
  PID Controller1/1 -> Saturation1/1, Integrator1/1
  Cos1/1 -> Product3/2
  Constant1/1 -> Sum3/2
  Product3/1 -> Sum2/1
  Sin1/1 -> Product2/2
  cos/1 -> Product3/1, Transfer Fcn1/1
  Integrator1/1 -> Sin1/1, Cos1/1, Sum3/1
  Sum2/1 -> PID Controller1/1, Scope1/1
  Product2/1 -> Sum2/2
  Sum3/1 -> Transfer Fcn4/1
  Transfer Fcn4/1 -> the/1

== matlab function saved3/全观测角速度闭环控制/w estimater/invpark ==
  data: u1 input; ua output; u2 input; ub output; t input
function [ua,ub] = fcn(u1,u2,t)
invPark=[cos(t) -sin(t);sin(t) cos(t)];
temp=invPark*[u1;u2];
ua=temp(1);
ub=temp(2);

== matlab function saved3/全观测角速度闭环控制/w estimater/clack ==
  data: ia input; iap output; ib input; ic input; ibe output
function [iap,ibe] = fcn(ia,ib,ic)
clack=2/3*[1 -1/2 -1/2;0 sqrt(3)/2 -sqrt(3)/2];
temp=clack*[ia;ib;ic];
iap=temp(1);
ibe=temp(2);

== matlab function saved3/全观测角速度闭环控制/w estimater/计算法求角速度 ==
  data: Ea input; y output; Eb input
function y = fcn(Ea,Eb)
phi=0.1;
y = sqrt(Ea^2+Eb^2)/phi*2/sqrt(3);

== matlab function saved3/全观测角速度闭环控制/w estimater/数据融合 ==
  data: cal input; y output; pll input
function y = fcn(cal,pll)
a=0.1;
h=0.95./(1+exp(-a*(cal+pll)/2));
y = h*(pll-cal)+cal;

== matlab function saved3/全观测角速度闭环控制/w estimater/MATLAB Function ==
  data: Ea input; y output; Eb input
function y = fcn(Ea,Eb)
if Ea^2+Eb^2<1e-1
    y=0;
else
    y = atan2(Ea,-Eb);
end

== matlab function saved3/全观测角速度闭环控制/软启动 ==
  data: t input; y output
function y = fcn(t)
t=t-0.05;
y = 0*(t<=0.05)+500*(t-0.05)*(0.05<t&&t<=0.35)+(250*(t-0.35)+150)*(0.35<t&&t<=0.55)+200*(t>0.55);

== matlab function saved3/离散化半成品/2pi 限制1 ==
  data: u input; y output
function y = fcn(u)

y = mod((u+pi),2*pi)-pi;

== matlab function saved3/全观测角速度闭环控制/controller/MATLAB Function ==
  data: wloop input; Vdirect input; Switch input; t input; out output
function out = fcn(wloop,Vdirect,Switch,t)
step1time=0.1;
step2time=0.2;
Ustart=1;
direction=1;
if t<step1time
    y=0;
else
    switch Switch
        case 0
            if t<step2time
                y=Ustart*direction;
            else
                y=wloop;
            end
        case 1
            y=Vdirect;
        otherwise
            y=0;
    end
end
out=y;

== matlab function saved3/离散化半成品/MATLAB Function7 ==
  data: t input; y output
function y = fcn(t)
t=t-0.05;
y = 0*(t<=0.05)+500*(t-0.05)*(0.05<t&&t<=0.35)+(250*(t-0.35)+150)*(0.35<t&&t<=0.55)+200*(t>0.55);

== matlab function saved3/离散化半成品/PSMS/PMSM dq/MATLAB Function ==
  data: u1 input; di1 output; u2 input; i1 input; i2 input; w input; di2 output
function [di1,di2] = fcn(u1,u2,i1,i2,w)
R=0.1; L1=1e-3; L2=1.4e-3;
phi=0.05;

A=[R/L1 -L2/L1*w;L1/L2*w R/L2];
Y=[1/L1 0;0 1/L2];
I=[i1;i2];
U=[u1;u2];

dI=-A*I+Y*U-phi*w*[0;1/L2];
di1=dI(1);
di2=dI(2);

== matlab function saved3/全观测角速度闭环控制/controller1/MATLAB Function ==
  data: wloop input; Vdirect input; Switch input; t input; out output
function out = fcn(wloop,Vdirect,Switch,t)
step1time=0.1;
step2time=0.2;
Ustart=1;
direction=1;
if t<step1time
    y=0;
else
    switch Switch
        case 0
            if t<step2time
                y=Ustart*direction;
            else
                y=wloop;
            end
        case 1
            y=Vdirect;
        otherwise
            y=0;
    end
end
out=y;
